simulink model "proyecto_a"  (R2023b)
settings: Solver=VariableStepAuto  StartTime=0.0  StopTime=0.1  RelTol=1e-3
undefined symbols (not defined in the file): test_ac1, test_ac2, test_ac3, test_am1, test_am2, test_am3, test_fc1, test_fc1_receptor, test_fc2, test_fc2_receptor, test_fc3, test_fc3_receptor, test_fm1, test_fm2, test_fm3, test_ts
libraries: commanapbnd3 x2
settings Model: Creator=RomaW11  LastModifiedBy=RomaW11

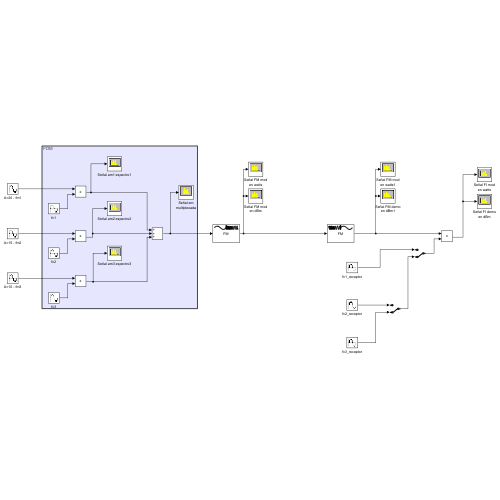
[thumbnail: Simulink's stored preview of the top-level diagram]
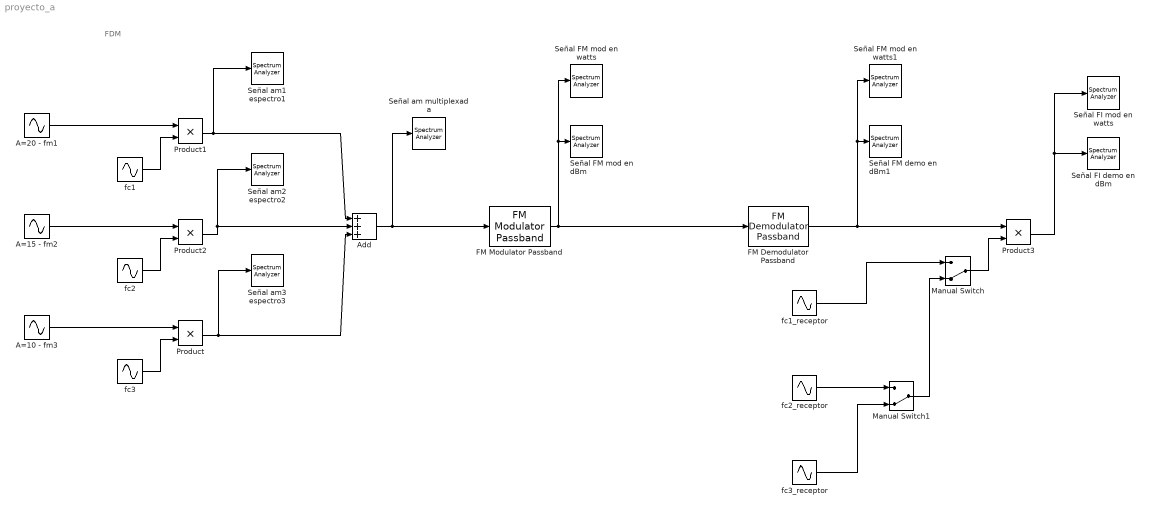
== system proyecto_a ==
  note: FDM
  A=10 - fm3 : Sin  Amplitude=test_am3  Frequency=2*pi*test_fm3  Phase=pi/2  SampleTime=test_ts
  A=15 - fm2 : Sin  Amplitude=test_am2  Frequency=2*pi*test_fm2  Phase=pi/2  SampleTime=test_ts
  A=20 - fm1 : Sin  Amplitude=test_am1  Frequency=2*pi*test_fm1  SampleTime=test_ts
  Add : Sum  Inputs=+++
  FM Demodulator Passband : commanapbnd3/FM Demodulator Passband  Fc=test_FM_mod  Ph=0  Kc=50  Ho=100
  FM Modulator Passband : commanapbnd3/FM Modulator Passband  Fc=test_FM_mod  Ph=0  Kc=50
  Manual Switch : ManualSwitch  CurrentSetting=0
  Manual Switch1 : ManualSwitch  CurrentSetting=0
  Product{,1..3} (4 alike) : Product
  Señal FI demo en dBm : SpectrumAnalyzer  WindowPosition=[1.000000,1.000000,1920.000000,1057.000000,]  ScopeFrameLocation=window  SampleRate=44.1e3  StartFrequency=20  StopFrequency=20e3  YLimits=[-106.50993919,36.77110611]  ShowLegend=on  SelectedToolstripTab=spectrumAnalyzerToolstrip.spectrumTab
      settings: OpenAtSimulationStart=off
  Señal FI mod en watts : SpectrumAnalyzer  WindowPosition=[1.000000,1.000000,1920.000000,1057.000000,]  ScopeFrameLocation=window  SampleRate=44.1e3  StartFrequency=20  StopFrequency=20e3  SpectrumUnits=Watts  YLimits=[-0.7814225,7.03280248]  ShowLegend=on  SelectedToolstripTab=spectrumAnalyzerToolstrip.spectrumTab
      settings: OpenAtSimulationStart=off
  Señal FM demo en dBm1 : SpectrumAnalyzer  WindowPosition=[1.000000,1.000000,1920.000000,1057.000000,]  ScopeFrameLocation=window  SampleRate=44.1e3  StartFrequency=20  StopFrequency=20e3  YLimits=[-84.49489701,58.22565386]  ShowLegend=on  SelectedToolstripTab=spectrumAnalyzerToolstrip.spectrumTab
      settings: OpenAtSimulationStart=off
  Señal FM mod en dBm : SpectrumAnalyzer  WindowPosition=[1.000000,1.000000,1920.000000,1057.000000,]  ScopeFrameLocation=window  SampleRate=44.1e3  StartFrequency=20  StopFrequency=20e3  YLimits=[-106.50993919,36.77110611]  ShowLegend=on  SelectedToolstripTab=spectrumAnalyzerToolstrip.spectrumTab
      settings: OpenAtSimulationStart=off
  Señal FM mod en watts : SpectrumAnalyzer  WindowPosition=[1.000000,1.000000,1920.000000,1057.000000,]  ScopeFrameLocation=window  SampleRate=44.1e3  StartFrequency=20  StopFrequency=20e3  SpectrumUnits=Watts  YLimits=[-0.02193866,0.19744797]  ShowLegend=on  SelectedToolstripTab=spectrumAnalyzerToolstrip.spectrumTab
      settings: OpenAtSimulationStart=off
  Señal FM mod en watts1 : SpectrumAnalyzer  WindowPosition=[1.000000,1.000000,1920.000000,1057.000000,]  ScopeFrameLocation=window  SampleRate=44.1e3  StartFrequency=20  StopFrequency=20e3  SpectrumUnits=Watts  YLimits=[-3.1064895,27.95840554]  ShowLegend=on  SelectedToolstripTab=spectrumAnalyzerToolstrip.spectrumTab
      settings: OpenAtSimulationStart=off
  Señal am multiplexada : SpectrumAnalyzer  WindowPosition=[1.000000,1.000000,1920.000000,1057.000000,]  ScopeFrameLocation=window  SampleRate=44.1e3  StartFrequency=20  StopFrequency=20e3  SpectrumUnits=Watts  YLimits=[-3.02841588,27.25574932]  ShowLegend=on  SelectedToolstripTab=spectrumAnalyzerToolstrip.spectrumTab
      settings: OpenAtSimulationStart=off
  Señal am1 espectro1 : SpectrumAnalyzer  WindowPosition=[1.000000,1.000000,1920.000000,1057.000000,]  ScopeFrameLocation=window  SampleRate=44.1e3  StartFrequency=20  StopFrequency=20e3  SpectrumUnits=Watts  YLimits=[-3.02836385,27.25527462]  ShowLegend=on  SelectedToolstripTab=spectrumAnalyzerToolstrip.spectrumTab
      settings: OpenAtSimulationStart=off
  Señal am2 espectro2 : SpectrumAnalyzer  WindowPosition=[1.000000,1.000000,1920.000000,1057.000000,]  ScopeFrameLocation=window  SampleRate=44.1e3  StartFrequency=20  StopFrequency=20e3  SpectrumUnits=Watts  YLimits=[-1.40886927,12.67982579]  ShowLegend=on  SelectedToolstripTab=spectrumAnalyzerToolstrip.spectrumTab
      settings: OpenAtSimulationStart=off
  Señal am3 espectro3 : SpectrumAnalyzer  WindowPosition=[1.000000,1.000000,1920.000000,1057.000000,]  ScopeFrameLocation=window  SampleRate=44.1e3  StartFrequency=20  StopFrequency=20e3  SpectrumUnits=Watts  YLimits=[-0.7176856,6.45917141]  ShowLegend=on  SelectedToolstripTab=spectrumAnalyzerToolstrip.spectrumTab
      settings: OpenAtSimulationStart=off
  fc1 : Sin  Amplitude=test_ac1  Frequency=2*pi*test_fc1  SampleTime=test_ts  VectorParams1D=off
  fc1_receptor : Sin  Frequency=2*pi*test_fc1_receptor  SampleTime=test_ts  VectorParams1D=off
  fc2 : Sin  Amplitude=test_ac2  Frequency=2*pi*test_fc2  Phase=pi/2  SampleTime=test_ts
  fc2_receptor : Sin  Frequency=2*pi*test_fc2_receptor  SampleTime=test_ts  VectorParams1D=off
  fc3 : Sin  Amplitude=test_ac3  Frequency=2*pi*test_fc3  Phase=pi/2  SampleTime=test_ts
  fc3_receptor : Sin  Frequency=2*pi*test_fc3_receptor  SampleTime=test_ts  VectorParams1D=off
  wires:
  Add/1 -> FM Modulator Passband/1, Señal am multiplexada/1
  A=20 - fm1/1 -> Product1/1
  A=15 - fm2/1 -> Product2/1
  fc3/1 -> Product/2
  fc1/1 -> Product1/2
  Product/1 -> Señal am3 espectro3/1, Add/3
  A=10 - fm3/1 -> Product/1
  Product2/1 -> Señal am2 espectro2/1, Add/2
  fc2/1 -> Product2/2
  Product1/1 -> Add/1, Señal am1 espectro1/1
  FM Modulator Passband/1 -> FM Demodulator Passband/1, Señal FM mod en watts/1, Señal FM mod en dBm/1
  FM Demodulator Passband/1 -> Product3/1, Señal FM mod en watts1/1, Señal FM demo en dBm1/1
  Manual Switch/1 -> Product3/2
  Manual Switch1/1 -> Manual Switch/2
  fc1_receptor/1 -> Manual Switch/1
  fc2_receptor/1 -> Manual Switch1/1
  fc3_receptor/1 -> Manual Switch1/2
  Product3/1 -> Señal FI mod en watts/1, Señal FI demo en dBm/1
